simulink model "unitVisualAqSurveillance"  (R2019b)
settings: Solver=VariableStepAuto  StartTime=0.0  StopTime=10.0  RelTol=1e-3
undefined symbols (not defined in the file or in its folder): ac1dyn_alt0_ft, ac1dyn_con, ac1dyn_lat0_rad, ac1dyn_lon0_rad, ac2dyn_alt0_ft, ac2dyn_con, ac2dyn_lat0_rad, ac2dyn_lon0_rad, ddh_ftps2, dh_ftps, dv_ftps2, e_ft, Edot_ftps, h_ft, hdot_ftps, latLonAltState, n_ft, Ndot_ftps, p_radps, phi_rad, phidot_radps, psi_rad, psidot_radps, q_radps, r_radps, theta_rad, thetadot_radps, v_ftps, vdot_fpss
libraries: simulink x14, VisualAqSurveillanceBlock_devAlt x1
(part 2 of 2)

== system unitVisualAqSurveillance/AC1 - Track Following/Follow Trajectory/Set State/Null AircraftState/Null LatLonAltMeasurement ==
  Bus Creator : BusCreator  Inputs='lat_rad','lon_rad','dlat_radps','dlon_radps','alt_ft','dalt_ftps'  OutDataTypeStr=Bus: LatLonAltMeasurement
  Constant{,1..5} (6 alike) : Constant  Value=0
  LLA : Outport  VectorParamsAs1DForOutWhenUnconnected=off
  wires:
  Constant1/1 -> Bus Creator/2  "lon_rad"
  Bus Creator/1 -> LLA/1
  Constant4/1 -> Bus Creator/5  "alt_ft"
  Constant5/1 -> Bus Creator/6  "dalt_ftps"
  Constant3/1 -> Bus Creator/4  "dlon_radps"
  Constant/1 -> Bus Creator/1  "lat_rad"
  Constant2/1 -> Bus Creator/3  "dlat_radps"

== system unitVisualAqSurveillance/AC2 - Track Following/Follow Trajectory/Set State/Null AircraftState/Null LatLonAltMeasurement ==
  Bus Creator : BusCreator  Inputs='lat_rad','lon_rad','dlat_radps','dlon_radps','alt_ft','dalt_ftps'  OutDataTypeStr=Bus: LatLonAltMeasurement
  Constant{,1..5} (6 alike) : Constant  Value=0
  LLA : Outport  VectorParamsAs1DForOutWhenUnconnected=off
  wires:
  Constant1/1 -> Bus Creator/2  "lon_rad"
  Bus Creator/1 -> LLA/1
  Constant4/1 -> Bus Creator/5  "alt_ft"
  Constant5/1 -> Bus Creator/6  "dalt_ftps"
  Constant3/1 -> Bus Creator/4  "dlon_radps"
  Constant/1 -> Bus Creator/1  "lat_rad"
  Constant2/1 -> Bus Creator/3  "dlat_radps"

== matlab function unitVisualAqSurveillance/AC1 - Track Following/Follow Trajectory/Set LLA /MATLAB Function ==
  data: e_ft input; n_ft input; u_ft input; v_ftps input; psi_rad input; theta_rad input; lat0 input; lat_rad output; lon0 input; h0 input; lon_rad output; dlat_radps output; dlon_radps output; alt_ft output; dalt_ftps output
function [lat_rad,lon_rad,dlat_radps,dlon_radps,alt_ft,dalt_ftps] = convertToLLA(e_ft,n_ft,u_ft,v_ftps,psi_rad,theta_rad,lat0,lon0,h0)
%#codegen

% WGS-84 ellipsoid constants
a = 2.09256*10^7;          %Semi-major axis (meters)
f = 1.0/298.257223563;  %Flattening
ecc_sq = f*(2.0-f);        %Eccentricity^2


% Ellipsoidal "radius"
er = a./sqrt(1-ecc_sq.*sin(lat0).^2);


% ECEF coordinates
x0 = (er + h0)*cos(lat0)*cos(lon0);
y0 = (er + h0)*cos(lat0)*sin(lon0);
z0 = (er.*(1-ecc_sq) + h0)*sin(lat0);


%% Rotation Matrix
posECEF0 = [x0;y0;z0];
% Compute the local Up unit vector
vHatU = posECEF0;
vHatU(3) = vHatU(3) ./ ((1-f)^2);
vHatU = vHatU ./ norm(vHatU);

% Compute the projection onto the local Up vector
pU = vHatU * vHatU';

% Compute the projection onto the local Tangent plane
pT = eye(size(pU)) - pU;

% Compute the local North unit vector
vHatZ = [0;0;1];
vHatN = pT * vHatZ;
vHatN = vHatN ./ norm(vHatN);

% Compute the local East unit vector
vHatE = cross(vHatN,vHatU);

% Compute ENU rotation matrix
rotMatENU = zeros(3,3);
rotMatENU(:,1) = vHatE;
rotMatENU(:,2) = vHatN;
rotMatENU(:,3) = vHatU;

tPosECEF = rotMatENU*[e_ft;n_ft;u_ft] + [x0;y0;z0];


%% ECEF to LLA
% WGS-84 derived parameters
b = (1-f).*a;                       %Semi-minor axis (meters)
ecc1_sq = (a.^2 - b.^2)./(a.^2);    %First eccentricity squared
ecc2_sq = (a.^2 - b.^2)./(b.^2);    %Second eccentricity squared


% Length of position vector in equatorial plane
rho = sqrt(tPosECEF(1).^2 + tPosECEF(2).^2);

% Auxillary angle
theta = atan( (tPosECEF(3).*a)./(rho.*b) );

lon_rad = atan2(tPosECEF(2),tPosECEF(1));
lat_rad = atan( (tPosECEF(3) + ecc2_sq.*b.*(sin(theta)).^3)./(rho - ecc1_sq.*a.*(cos(theta)).^3) );

ewRadCurv = a./sqrt(1-ecc1_sq.*sin(lat_rad).^2);

alt_ft = (rho./cos(lat_rad)) - ewRadCurv;


%% Velocities - Project 1 sec into future and use to estimate
dalt_ftps = v_ftps*sin(theta_rad); % Assume about the same


tPosECEF_1sec = rotMatENU*[e_ft+v_ftps*sin(theta_rad)*sin(psi_rad);...
                           n_ft+v_ftps*sin(theta_rad)*cos(psi_rad);...
                           u_ft] + ...
                           [x0;y0;z0];

% Length of position vector in equatorial plane
rho = sqrt(tPosECEF_1sec(1).^2 + tPosECEF_1sec(2).^2);

% Auxillary angle
theta = atan( (tPosECEF_1sec(3).*a)./(rho.*b) );

lon_rad_1sec = atan2(tPosECEF_1sec(2),tPosECEF_1sec(1));
lat_rad_1sec = atan( (tPosECEF_1sec(3) + ecc2_sq.*b.*(sin(theta)).^3)./(rho - ecc1_sq.*a.*(cos(theta)).^3) );

dlat_radps = lat_rad_1sec - lat_rad;
dlon_radps = lon_rad_1sec - lon_rad;
end

== matlab function unitVisualAqSurveillance/AC2 - Track Following/Follow Trajectory/Set LLA /MATLAB Function ==
  data: e_ft input; n_ft input; u_ft input; v_ftps input; psi_rad input; theta_rad input; lat0 input; lat_rad output; lon0 input; h0 input; lon_rad output; dlat_radps output; dlon_radps output; alt_ft output; dalt_ftps output
function [lat_rad,lon_rad,dlat_radps,dlon_radps,alt_ft,dalt_ftps] = convertToLLA(e_ft,n_ft,u_ft,v_ftps,psi_rad,theta_rad,lat0,lon0,h0)
%#codegen

% WGS-84 ellipsoid constants
a = 2.09256*10^7;          %Semi-major axis (meters)
f = 1.0/298.257223563;  %Flattening
ecc_sq = f*(2.0-f);        %Eccentricity^2


% Ellipsoidal "radius"
er = a./sqrt(1-ecc_sq.*sin(lat0).^2);


% ECEF coordinates
x0 = (er + h0)*cos(lat0)*cos(lon0);
y0 = (er + h0)*cos(lat0)*sin(lon0);
z0 = (er.*(1-ecc_sq) + h0)*sin(lat0);


%% Rotation Matrix
posECEF0 = [x0;y0;z0];
% Compute the local Up unit vector
vHatU = posECEF0;
vHatU(3) = vHatU(3) ./ ((1-f)^2);
vHatU = vHatU ./ norm(vHatU);

% Compute the projection onto the local Up vector
pU = vHatU * vHatU';

% Compute the projection onto the local Tangent plane
pT = eye(size(pU)) - pU;

% Compute the local North unit vector
vHatZ = [0;0;1];
vHatN = pT * vHatZ;
vHatN = vHatN ./ norm(vHatN);

% Compute the local East unit vector
vHatE = cross(vHatN,vHatU);

% Compute ENU rotation matrix
rotMatENU = zeros(3,3);
rotMatENU(:,1) = vHatE;
rotMatENU(:,2) = vHatN;
rotMatENU(:,3) = vHatU;

tPosECEF = rotMatENU*[e_ft;n_ft;u_ft] + [x0;y0;z0];


%% ECEF to LLA
% WGS-84 derived parameters
b = (1-f).*a;                       %Semi-minor axis (meters)
ecc1_sq = (a.^2 - b.^2)./(a.^2);    %First eccentricity squared
ecc2_sq = (a.^2 - b.^2)./(b.^2);    %Second eccentricity squared


% Length of position vector in equatorial plane
rho = sqrt(tPosECEF(1).^2 + tPosECEF(2).^2);

% Auxillary angle
theta = atan( (tPosECEF(3).*a)./(rho.*b) );

lon_rad = atan2(tPosECEF(2),tPosECEF(1));
lat_rad = atan( (tPosECEF(3) + ecc2_sq.*b.*(sin(theta)).^3)./(rho - ecc1_sq.*a.*(cos(theta)).^3) );

ewRadCurv = a./sqrt(1-ecc1_sq.*sin(lat_rad).^2);

alt_ft = (rho./cos(lat_rad)) - ewRadCurv;


%% Velocities - Project 1 sec into future and use to estimate
dalt_ftps = v_ftps*sin(theta_rad); % Assume about the same


tPosECEF_1sec = rotMatENU*[e_ft+v_ftps*sin(theta_rad)*sin(psi_rad);...
                           n_ft+v_ftps*sin(theta_rad)*cos(psi_rad);...
                           u_ft] + ...
                           [x0;y0;z0];

% Length of position vector in equatorial plane
rho = sqrt(tPosECEF_1sec(1).^2 + tPosECEF_1sec(2).^2);

% Auxillary angle
theta = atan( (tPosECEF_1sec(3).*a)./(rho.*b) );

lon_rad_1sec = atan2(tPosECEF_1sec(2),tPosECEF_1sec(1));
lat_rad_1sec = atan( (tPosECEF_1sec(3) + ecc2_sq.*b.*(sin(theta)).^3)./(rho - ecc1_sq.*a.*(cos(theta)).^3) );

dlat_radps = lat_rad_1sec - lat_rad;
dlon_radps = lon_rad_1sec - lon_rad;
end
